simulink model "LQR_vehicle_dynamic_model"  (R2021b)
settings: Solver=ode45  StartTime=0.0  StopTime=60  RelTol=0.1
model workspace (MAT data in the model file):
  k1 = [0.316227766019 0.316227766017 0.316227766017 0.316227766017 0.316227766017 0.316227766017 0.316227766017 0.316227766017 0.316227766017 0.316227766017 0.316227766017 0.316227766017 ... (5000 elements, 1x5000)]
  k2 = [0.000301883202587 0.000603764374018 0.000905641483218 0.00120751249925 0.00150937539142 0.00181122812931 0.00211306868289 0.00241489502258 0.00271670511931 0.00301849694462 0.00332026847071 0.00362201767054 ... (5000 elements, 1x5000)]
  k3 = [0.945396449835 0.945404346198 0.945417506418 0.945435929946 0.945459615988 0.945488563526 0.945522771323 0.945562237918 0.945606961617 0.945656940508 0.945712172453 0.945772655093 ... (5000 elements, 1x5000)]
  k4 = [0.000322785568317 0.000645569647506 0.000968350748438 0.00129112738198 0.00161389805896 0.00193666129021 0.00225941558652 0.00258215945866 0.00290489141734 0.00322760997326 0.00355031363705 0.00387300091929 ... (5000 elements, 1x5000)]
  kappar = [0 0 0 0 0 0 0 0 0 0 0 0 ... (4802 elements, 1x4802)]
  thetar = [0 0 0 0 0 0 0 0 0 0 0 0 ... (4802 elements, 1x4802)]
  xr = [0.0501253132832 0.100250626566 0.15037593985 0.200501253133 0.250626566416 0.300751879699 0.350877192982 0.401002506266 0.451127819549 0.501253132832 0.551378446115 0.601503759398 ... (4802 elements, 1x4802)]
  yr = [0 0 0 0 0 0 0 0 0 0 0 0 ... (4802 elements, 1x4802)]
libraries: simulink x1
(part 1 of 2)
settings Model: Creator=JHD  LastModifiedBy=Jing
settings SolverCC: AlgebraicLoopSolver=TrustRegion
settings DebuggingCC: SFMachineParentedDataDiag=warning  UnderSpecifiedDimensionMsg=warning

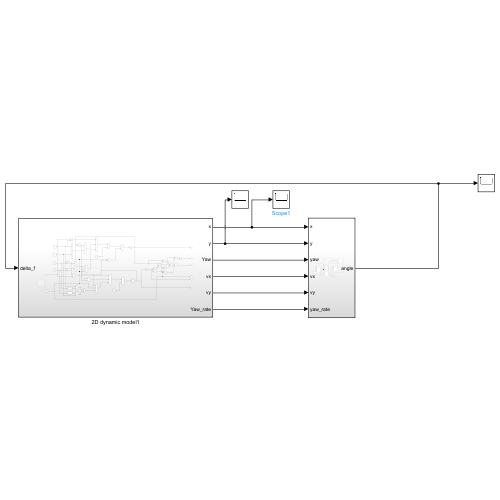
[thumbnail: Simulink's stored preview of the top-level diagram]
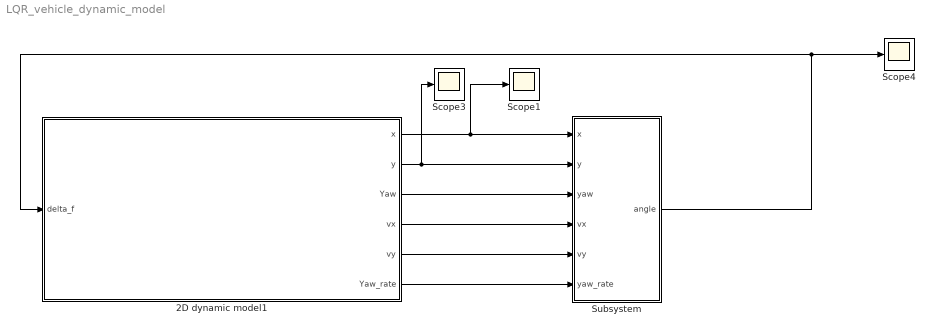
== system LQR_vehicle_dynamic_model ==
  2D dynamic model1 : Subsystem
  Scope1 : Scope
  Scope3 : Scope
  Scope4 : Scope
  Subsystem : Subsystem
  wires:
  2D dynamic model1/1(x) -> Scope1/1, Subsystem/1(x)
  2D dynamic model1/2(y) -> Scope3/1, Subsystem/2(y)
  2D dynamic model1/3(Yaw) -> Subsystem/3(yaw)
  2D dynamic model1/4(vx) -> Subsystem/4(vx)
  2D dynamic model1/5(vy) -> Subsystem/5(vy)
  2D dynamic model1/6(Yaw_rate) -> Subsystem/6(yaw_rate)
  Subsystem/1(angle) -> 2D dynamic model1/1(delta_f), Scope4/1
